simulink model "ECU_ABS_Model"  (R2025a)
settings: Solver=ode4  StartTime=0.0  StopTime=26  FixedStep=0.0001  RelTol=1e-3  EnableMultiTasking=on
libraries: arduinolib x1, SignalEditorBlockLib x1
settings Model: SILPILModeSetting=veronly  ExtModeTrigDuration=2  Creator=ec97883  LastModifiedBy=Dell
settings SolverCC: AutoInsertRateTranBlk=on
settings OptimizationCC: EnhancedBackFolding=on  PassReuseOutputArgsAs=Individual arguments  ZeroExternalMemoryAtStartup=off  ZeroInternalMemoryAtStartup=off  MaxStackSize=64  OptimizeBlockOrder=speed  DifferentSizesBufferReuse=on  OptimizationCustomize=off  EfficientTunableParamExpr=on
settings DebuggingCC: ParameterTunabilityLossMsg=error
settings HardwareCC: ProdBitPerInt=16.0  ProdBitPerPointer=16.0  ProdBitPerSizeT=16.0  ProdBitPerPtrDiffT=16.0  ProdLargestAtomicFloat=None  ProdWordSize=8.0  ProdHWDeviceType=Atmel->AVR  UseEmbeddedCoderFeatures=off
settings SFSimCC: MATLABDynamicMemAlloc=off
settings RTWCC: SystemTargetFile=ert.tlc  HardwareBoard=Arduino Uno  TemplateMakefile=ert_default_tmf  Toolchain=Arduino AVR  BuildConfiguration=Faster Runs  Description=Embedded Coder
settings CodeAppCC: ForceParamTrailComments=on  IgnoreCustomStorageClasses=off  OperatorAnnotations=on  SimulinkDataObjDesc=on  SFDataObjDesc=on  InsertBlockDesc=on
settings ERTTargetCC: ExtModeTransport=3.0  ExtModeAutomaticAllocSize=off  ExtModeStaticAllocSize=250.0  InlinedParameterPlacement=Hierarchical  SupportContinuousTime=on  SupportNonInlinedSFcns=on  SupportVariableSizeSignals=on

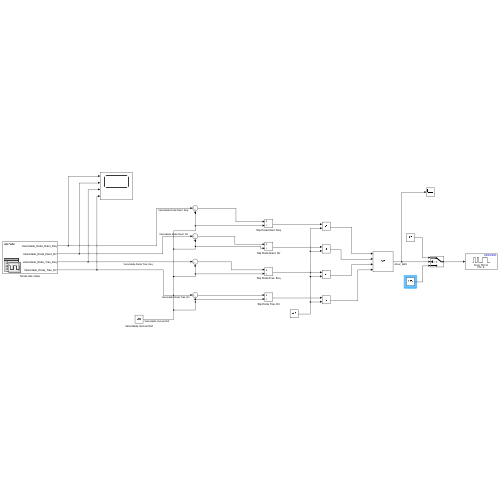
[thumbnail: Simulink's stored preview of the top-level diagram]
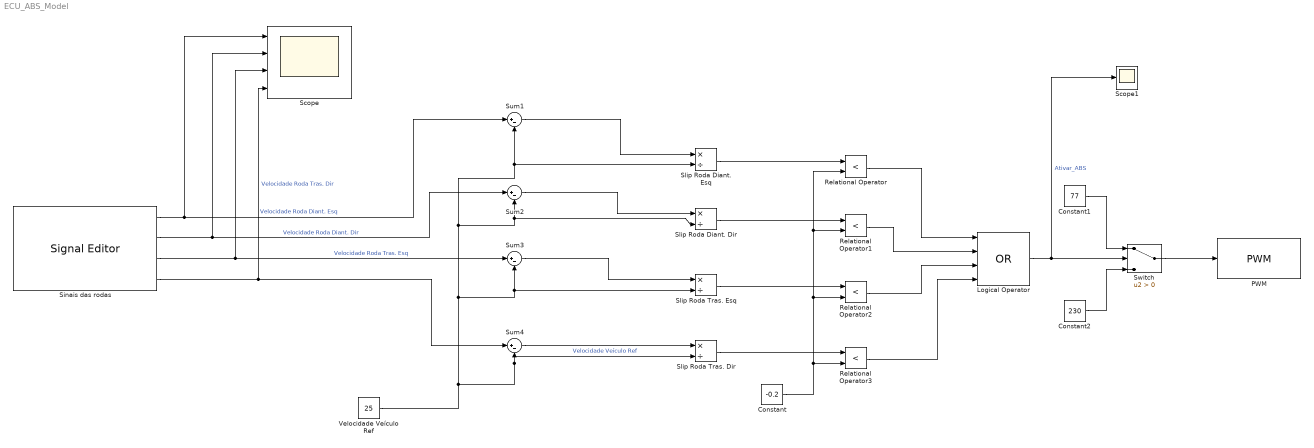
== system ECU_ABS_Model ==
  Constant : Constant  Value=-0.2  OutDataTypeStr=double
  Constant1 : Constant  Value=77
  Constant2 : Constant  Value=230
  Logical Operator : Logic  Operator=OR  Inputs=4  AllPortsSameDT=off  OutDataTypeStr=boolean
  PWM : arduinolib/PWM  pinNumber=9  frequencyType=Specify  desiredFrequency=50  achievableFrequency=50
      settings: LibrarySourceBlock=gizmoLibrary/Arduino Utilities/PWM
  Relational Operator{,1..3} (4 alike) : RelationalOperator  Operator=<  OutDataTypeStr=boolean  RndMeth=Simplest  InputSameDT=off
  Scope : Scope  NumInputPorts=4
      settings: ActiveDisplayYMinimum=-2.4999999999999996  ActiveDisplayYMaximum=22.5
  Scope1 : Scope
      settings: ActiveDisplayYMinimum=-0.12499999999999997  ActiveDisplayYMaximum=1.125
  Sinais das rodas : SignalEditorBlockLib/Signal Editor  FileName=Sinais_das_Rodas.mat  ActiveScenario=Scenario  ActiveSignal=Velocidade_Roda_Diant_Dir  IsBus=off  OutputBusObjectStr=Bus: BusObject  SampleTime=0  Interpolate=off  ZeroCross=off  OutputAfterFinalValue=Setting to zero  Unit=inherit  PreserveSignalName=on  ApplySigPropsToAllScenarios=on  ApplySigPropsToAllSignals=off  SignalPropertySource=Dialog parameters
  Slip Roda Diant. Dir : Product  Inputs=*/  OutDataTypeStr=double
  Slip Roda Diant. Esq : Product  Inputs=*/  OutDataTypeStr=double
  Slip Roda Tras. Dir : Product  Inputs=*/  OutDataTypeStr=double
  Slip Roda Tras. Esq : Product  Inputs=*/  OutDataTypeStr=double
  Sum{1..4} (4 alike) : Sum  Inputs=|+-  OutDataTypeStr=double
  Switch : Switch  Criteria=u2 > Threshold  SaturateOnIntegerOverflow=off  InputSameDT=off
  Velocidade Veículo Ref : Constant  Value=25  OutDataTypeStr=double
  wires:
  Sinais das rodas/1 -> Scope/1, Sum1/1  "Velocidade Roda Diant. Esq"
  Sinais das rodas/2 -> Scope/2, Sum2/1  "Velocidade Roda Diant. Dir"
  Sinais das rodas/3 -> Scope/3, Sum3/1  "Velocidade Roda Tras. Esq"
  Sinais das rodas/4 -> Scope/4, Sum4/1  "Velocidade Roda Tras. Dir"
  Sum1/1 -> Slip Roda Diant. Esq/1
  Sum2/1 -> Slip Roda Diant. Dir/1
  Sum3/1 -> Slip Roda Tras. Esq/1
  Sum4/1 -> Slip Roda Tras. Dir/1
  Slip Roda Diant. Esq/1 -> Relational Operator/1
  Slip Roda Diant. Dir/1 -> Relational Operator1/1
  Slip Roda Tras. Esq/1 -> Relational Operator2/1
  Slip Roda Tras. Dir/1 -> Relational Operator3/1
  Constant/1 -> Relational Operator3/2, Relational Operator2/2, Relational Operator1/2, Relational Operator/2
  Relational Operator/1 -> Logical Operator/1
  Relational Operator1/1 -> Logical Operator/2
  Relational Operator2/1 -> Logical Operator/3
  Relational Operator3/1 -> Logical Operator/4
  Velocidade Veículo Ref/1 -> Slip Roda Tras. Dir/2, Sum4/2, Sum3/2, Slip Roda Tras. Esq/2, Slip Roda Diant. Dir/2, Sum2/2, Slip Roda Diant. Esq/2, Sum1/2  "Velocidade Veículo Ref"
  Logical Operator/1 -> Switch/2, Scope1/1  "Ativar_ABS"
  Switch/1 -> PWM/1
  Constant1/1 -> Switch/1
  Constant2/1 -> Switch/3
